simulink model "EngPrt_PrtLimMech"  (R2018a)
settings: configuration reference "cs_ert" (kept outside this file)
model workspace (MAT data in the model file):
  EngPrt_PrtLimMech_DT = 10
values from neighbouring files (symbols this model uses):
  EngPrt_facTrqLimCor_MAP = 1.0 1.0 1.0 1.0 1.0 1.0 1.0 1.0 1.0 1.0 1.0 1.0 1.0 1.0 1.0 1.0 1.0 1.0 1.0 1.0 1.0 1.0 1.0 1.0 1.0 1.0 1.0 1.0 1.0 1.0 1.0 1.0 1.0 1.0 1.0 1.0 1.0 1.0 1.0 1.0 1.0 1.0 1.0 1.0 1.0 1.0 1.0 1.0 1.0 1.0 1.0 1.0 1.0 1.0 1.0 1.0 1.0 1.0 1.0 1.0 1.0 1.0 1.0 1.0 1.0 1.0 1.0 1.0 1.0 1.0 1.0 1.0 1.0 1.0 1.0 1.0 1.0 1.0 1.0 1.0 1.0 1.0 1.0 1.0 1.0 1.0 1.0 1.0 1.0 1.0 1.0 1.0 1.0 1.0 1.0 1.0 1.0 1.0 1.0 1.0    [EngPrt_PrtLimMech.sldd]
  EngPrt_facTrqLimCor_MAPX : value not decoded    [EngPrt_PrtLimMech.sldd]
  EngPrt_facTrqLimCor_MAPY : value not decoded    [EngPrt_PrtLimMech.sldd]
  EngPrt_qLim_CUR : value not decoded    [EngPrt_PrtLimMech.sldd]
  EngPrt_qLim_CURX = 100.0 345.83333333333337 591.66666666666674 837.5 1083.3333333333335 1329.1666666666667 1575.0 1820.8333333333333 2066.666666666667 2312.5 2558.3333333333335 2804.1666666666665 3050.0 3295.8333333333335 3541.6666666666665 3787.5 4033.3333333333335 4279.166666666667 4525.0 4770.833333333333 5016.666666666667 5262.5 5508.333333333333 5754.166666666667 6000.0    [EngPrt_PrtLimMech.sldd]
  EngPrt_RmpLimNErrNeg_C = 10.0    [EngPrt_PrtLimMech.sldd]
  EngPrt_RmpLimNErrPos_C = 10.0    [EngPrt_PrtLimMech.sldd]
  EngPrt_swtLimCorType_C = 0    [EngPrt_PrtLimMech.sldd]
  EngPrt_swtTrq_C = 0.0    [EngPrt_PrtLimMech.sldd]
  EngPrt_trqLim_CUR : value not decoded    [EngPrt_PrtLimMech.sldd]
  EngPrt_trqLim_CURX : value not decoded    [EngPrt_PrtLimMech.sldd]
  EngPrt_trqLimAPSCor_MAP = 0.0 0.0 0.0 0.0 0.0 0.0 0.0 0.0 0.0 0.0 0.0 0.0 0.0 0.0 0.0 0.0 0.0 0.0 0.0 0.0 0.0 0.0 0.0 0.0 0.0 0.0 0.0 0.0 0.0 0.0 0.0 0.0 0.0 0.0 0.0 0.0 0.0 0.0 0.0 0.0 0.0 0.0 0.0 0.0 0.0 0.0 0.0 0.0 0.0 0.0 0.0 0.0 0.0 0.0 0.0 0.0 0.0 0.0 0.0 0.0 0.0 0.0 0.0 0.0 0.0 0.0 0.0 0.0 0.0 0.0 0.0 0.0 0.0 0.0 0.0 0.0 0.0 0.0 0.0 0.0 0.0 0.0 0.0 0.0 0.0 0.0 0.0 0.0 0.0 0.0 0.0 0.0 0.0 0.0 0.0 0.0 0.0 0.0 0.0 0.0    [EngPrt_PrtLimMech.sldd]
  EngPrt_trqLimAPSCor_MAPX : value not decoded    [EngPrt_PrtLimMech.sldd]
  EngPrt_trqLimAPSCor_MAPY : value not decoded    [EngPrt_PrtLimMech.sldd]
  EngPrt_trqLimEngTempCor_MAP = 0.0 0.0 0.0 0.0 0.0 0.0 0.0 0.0 0.0 0.0 0.0 0.0 0.0 0.0 0.0 0.0 0.0 0.0 0.0 0.0 0.0 0.0 0.0 0.0 0.0 0.0 0.0 0.0 0.0 0.0 0.0 0.0 0.0 0.0 0.0 0.0 0.0 0.0 0.0 0.0 0.0 0.0 0.0 0.0 0.0 0.0 0.0 0.0 0.0 0.0 0.0 0.0 0.0 0.0 0.0 0.0 0.0 0.0 0.0 0.0 0.0 0.0 0.0 0.0 0.0 0.0 0.0 0.0 0.0 0.0 0.0 0.0 0.0 0.0 0.0 0.0 0.0 0.0 0.0 0.0 0.0 0.0 0.0 0.0 0.0 0.0 0.0 0.0 0.0 0.0 0.0 0.0 0.0 0.0 0.0 0.0 0.0 0.0 0.0 0.0    [EngPrt_PrtLimMech.sldd]
  EngPrt_trqLimEngTempCor_MAPX : value not decoded    [EngPrt_PrtLimMech.sldd]
  EngPrt_trqLimEngTempCor_MAPY : value not decoded    [EngPrt_PrtLimMech.sldd]
  EngPrt_trqNLim_CUR : value not decoded    [EngPrt_PrtLimMech.sldd]
  EngPrt_trqNLim_CURX : value not decoded    [EngPrt_PrtLimMech.sldd]
  EngPrt_trqNLimSpr_CUR : value not decoded    [EngPrt_PrtLimMech.sldd]
  EngPrt_trqNLimSpr_CURX : value not decoded    [EngPrt_PrtLimMech.sldd]
undefined symbols (not defined in the file or in its folder): Switch
libraries: sllib x1
settings Model: DataDictionary=EngPrt_PrtLimMech.sldd  Creator=zhoutinglin  LastModifiedBy=zhoutinglin

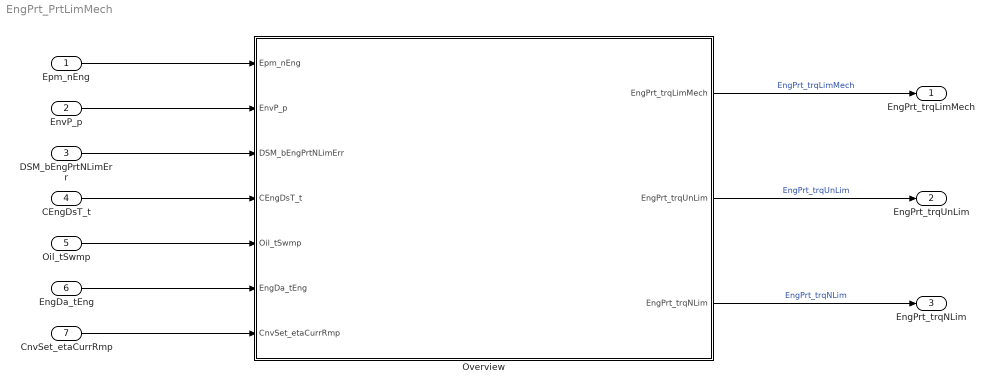
== system EngPrt_PrtLimMech ==
  Epm_nEng : Inport  Description=Engine speed  OutMin=0  OutMax=6000  OutDataTypeStr=ERPM  Unit=rpm  PortDimensions=[1 1]
  EnvP_p : Inport  Description=Barometric pressure  Port=2  OutMin=0  OutMax=300  OutDataTypeStr=Press_kpa  Unit=kPa  PortDimensions=[1 1]
  DSM_bEngPrtNLimErr : Inport  Description=Activation of additional engine speed limitation  Port=3  OutMin=0  OutMax=1  OutDataTypeStr=boolean  PortDimensions=[1 1]
  CEngDsT_t : Inport  Description=engine coolant temperature after filter  Port=4  OutMin=-200  OutMax=200  OutDataTypeStr=Temp_C  Unit=deg  PortDimensions=[1 1]
  Oil_tSwmp : Inport  Description=Oil temperature in oil sump  Port=5  OutMin=-50  OutMax=200  OutDataTypeStr=Temp_C  Unit=deg  PortDimensions=[1 1]
  EngDa_tEng : Inport  Description=Engine temperature  Port=6  OutMin=-1000  OutMax=1000  OutDataTypeStr=Temp_C  Unit=deg  PortDimensions=[1 1]
  CnvSet_etaCurrRmp : Inport  Description=Conversion efficiency corresponding to CnvSet_qSet  Port=7  OutMin=0  OutMax=100  OutDataTypeStr=Effcy  Unit=Nm/(mg/hub)  PortDimensions=[1 1]
  Overview : Subsystem
  EngPrt_trqLimMech : Outport
  EngPrt_trqUnLim : Outport  Port=2
  EngPrt_trqNLim : Outport  Port=3
  wires:
  Epm_nEng/1 -> Overview/1(Epm_nEng)
  EnvP_p/1 -> Overview/2(EnvP_p)
  DSM_bEngPrtNLimErr/1 -> Overview/3(DSM_bEngPrtNLimErr)
  CEngDsT_t/1 -> Overview/4(CEngDsT_t)
  Oil_tSwmp/1 -> Overview/5(Oil_tSwmp)
  EngDa_tEng/1 -> Overview/6(EngDa_tEng)
  CnvSet_etaCurrRmp/1 -> Overview/7(CnvSet_etaCurrRmp)
  Overview/1(EngPrt_trqLimMech) -> EngPrt_trqLimMech/1  "EngPrt_trqLimMech"
  Overview/2(EngPrt_trqUnLim) -> EngPrt_trqUnLim/1  "EngPrt_trqUnLim"
  Overview/3(EngPrt_trqNLim) -> EngPrt_trqNLim/1  "EngPrt_trqNLim"

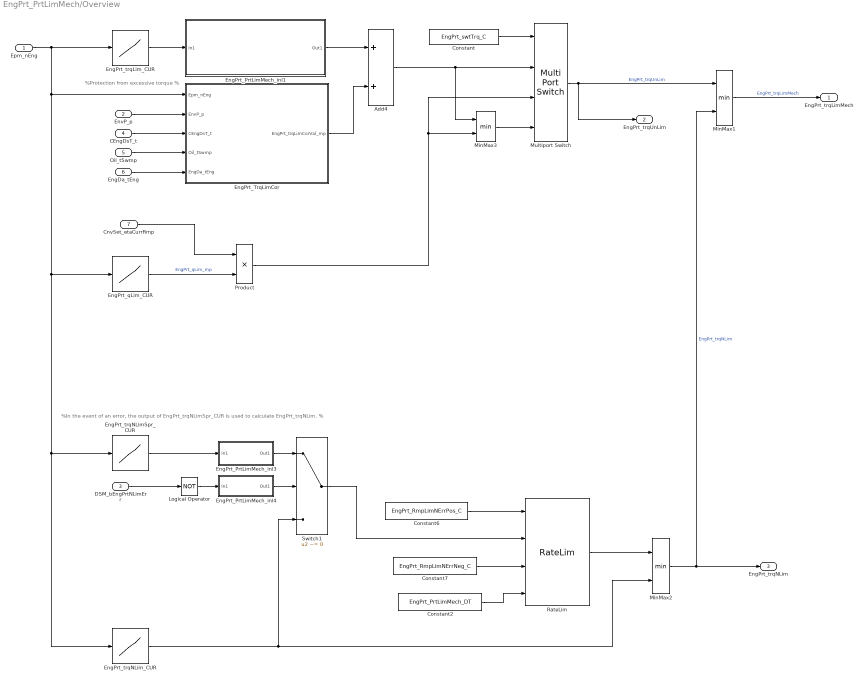
== system EngPrt_PrtLimMech/Overview ==
  note: %Protection from excessive torque %
  note: %In the event of an error, the output of EngPrt_trqNLimSpr_CUR is used to calculate EngPrt_trqNLim. %
  Epm_nEng : Inport  Tag=rpm
  EnvP_p : Inport  Tag=kPa  Port=2
  DSM_bEngPrtNLimErr : Inport  Port=3
  CEngDsT_t : Inport  Tag=deg  Port=4
  Oil_tSwmp : Inport  Tag=deg  Port=5
  EngDa_tEng : Inport  Tag=deg  Port=6
  CnvSet_etaCurrRmp : Inport  Tag=Nm/(mg/hub)  Port=7
  Add4 : Sum  InputSameDT=on
  Constant : Constant  Value=EngPrt_swtTrq_C
  Constant2 : Constant  Value=EngPrt_PrtLimMech_DT  OutDataTypeStr=Inherit: Inherit via back propagation
  Constant6 : Constant  Value=EngPrt_RmpLimNErrPos_C
  Constant7 : Constant  Value=EngPrt_RmpLimNErrNeg_C
  EngPrt_PrtLimMech_inl1 : Subsystem
  EngPrt_PrtLimMech_inl3 : Subsystem
  EngPrt_PrtLimMech_inl4 : Subsystem
  EngPrt_TrqLimCor : Subsystem
  EngPrt_qLim_CUR : Lookup_n-D  NumberOfTableDimensions=1  BreakpointsForDimension1=EngPrt_qLim_CURX  BreakpointsForDimension2=[1:3]  IndexSearchMethod=Linear search  Table=EngPrt_qLim_CUR  ExtrapMethod=Clip  InternalRulePriority=Speed  OutDataTypeStr=Inherit: Inherit via back propagation  RndMeth=Simplest  SaturateOnIntegerOverflow=on
  EngPrt_trqLim_CUR : Lookup_n-D  NumberOfTableDimensions=1  BreakpointsForDimension1=EngPrt_trqLim_CURX  BreakpointsForDimension2=[1:3]  IndexSearchMethod=Linear search  Table=EngPrt_trqLim_CUR  ExtrapMethod=Clip  InternalRulePriority=Speed  OutDataTypeStr=Inherit: Inherit via back propagation  RndMeth=Simplest  SaturateOnIntegerOverflow=on
  EngPrt_trqNLimSpr_CUR : Lookup_n-D  NumberOfTableDimensions=1  BreakpointsForDimension1=EngPrt_trqNLimSpr_CURX  BreakpointsForDimension2=[1:3]  IndexSearchMethod=Linear search  Table=EngPrt_trqNLimSpr_CUR  ExtrapMethod=Clip  InternalRulePriority=Speed  OutDataTypeStr=Inherit: Inherit via back propagation  RndMeth=Simplest  SaturateOnIntegerOverflow=on
  EngPrt_trqNLim_CUR : Lookup_n-D  NumberOfTableDimensions=1  BreakpointsForDimension1=EngPrt_trqNLim_CURX  BreakpointsForDimension2=[1:3]  IndexSearchMethod=Linear search  Table=EngPrt_trqNLim_CUR  ExtrapMethod=Clip  InternalRulePriority=Speed  OutDataTypeStr=Inherit: Inherit via back propagation  RndMeth=Simplest  SaturateOnIntegerOverflow=on
  Logical Operator : Logic  Operator=NOT  AllPortsSameDT=off  OutDataTypeStr=boolean
  MinMax1 : MinMax  Inputs=2  InputSameDT=on
  MinMax2 : MinMax  Inputs=2  InputSameDT=on
  MinMax3 : MinMax  Inputs=2  InputSameDT=on
  Multiport Switch : MultiPortSwitch  DataPortOrder=Zero-based contiguous  zeroidx=on  OutDataTypeStr=Inherit: Inherit via back propagation  InputSameDT=on
  Product : Product  OutDataTypeStr=Inherit: Inherit via back propagation  SaturateOnIntegerOverflow=on
  RateLim : sllib/RateLim
      settings: SourceProductName=sllib
  Switch1 : Switch  Criteria=u2 ~= 0  InputSameDT=on
  EngPrt_trqLimMech : Outport  Tag=Nm
  EngPrt_trqUnLim : Outport  Tag=Nm  Port=2
  EngPrt_trqNLim : Outport  Tag=Nm  Port=3
  wires:
  Add4/1 -> Multiport Switch/2, MinMax3/1
  Multiport Switch/1 -> EngPrt_trqUnLim/1, MinMax1/1  "EngPrt_trqUnLim"
  EngPrt_trqNLim_CUR/1 -> MinMax2/2, Switch1/3
  CnvSet_etaCurrRmp/1 -> Product/1
  EngPrt_qLim_CUR/1 -> Product/2  "EngPrt_qLim_mp"
  Product/1 -> Multiport Switch/3, MinMax3/2
  MinMax2/1 -> MinMax1/2, EngPrt_trqNLim/1  "EngPrt_trqNLim"
  RateLim/1 -> MinMax2/1
  Constant2/1 -> RateLim/4
  Constant/1 -> Multiport Switch/1
  EngPrt_PrtLimMech_inl4/1(Out1) -> Switch1/2
  MinMax3/1 -> Multiport Switch/4
  Oil_tSwmp/1 -> EngPrt_TrqLimCor/4(Oil_tSwmp)
  EngPrt_PrtLimMech_inl1/1(Out1) -> Add4/1
  MinMax1/1 -> EngPrt_trqLimMech/1  "EngPrt_trqLimMech"
  EngPrt_trqNLimSpr_CUR/1 -> EngPrt_PrtLimMech_inl3/1(In1)
  DSM_bEngPrtNLimErr/1 -> Logical Operator/1
  Switch1/1 -> RateLim/2
  EngPrt_PrtLimMech_inl3/1(Out1) -> Switch1/1
  Constant7/1 -> RateLim/3
  Constant6/1 -> RateLim/1
  EngDa_tEng/1 -> EngPrt_TrqLimCor/5(EngDa_tEng)
  EngPrt_TrqLimCor/1(EngPrt_trqLimCorVal_mp) -> Add4/2
  EnvP_p/1 -> EngPrt_TrqLimCor/2(EnvP_p)
  CEngDsT_t/1 -> EngPrt_TrqLimCor/3(CEngDsT_t)
  Logical Operator/1 -> EngPrt_PrtLimMech_inl4/1(In1)
  EngPrt_trqLim_CUR/1 -> EngPrt_PrtLimMech_inl1/1(In1)
  Epm_nEng/1 -> EngPrt_qLim_CUR/1, EngPrt_trqNLim_CUR/1, EngPrt_trqNLimSpr_CUR/1, EngPrt_TrqLimCor/1(Epm_nEng), EngPrt_trqLim_CUR/1

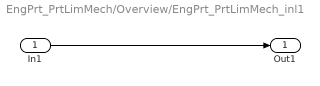
== system EngPrt_PrtLimMech/Overview/EngPrt_PrtLimMech_inl1 ==
  In1 : Inport
  Out1 : Outport
  wires:
  In1/1 -> Out1/1

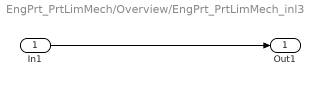
== system EngPrt_PrtLimMech/Overview/EngPrt_PrtLimMech_inl3 ==
  In1 : Inport
  Out1 : Outport
  wires:
  In1/1 -> Out1/1

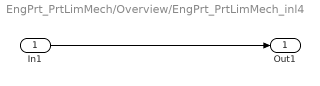
== system EngPrt_PrtLimMech/Overview/EngPrt_PrtLimMech_inl4 ==
  In1 : Inport
  Out1 : Outport
  wires:
  In1/1 -> Out1/1

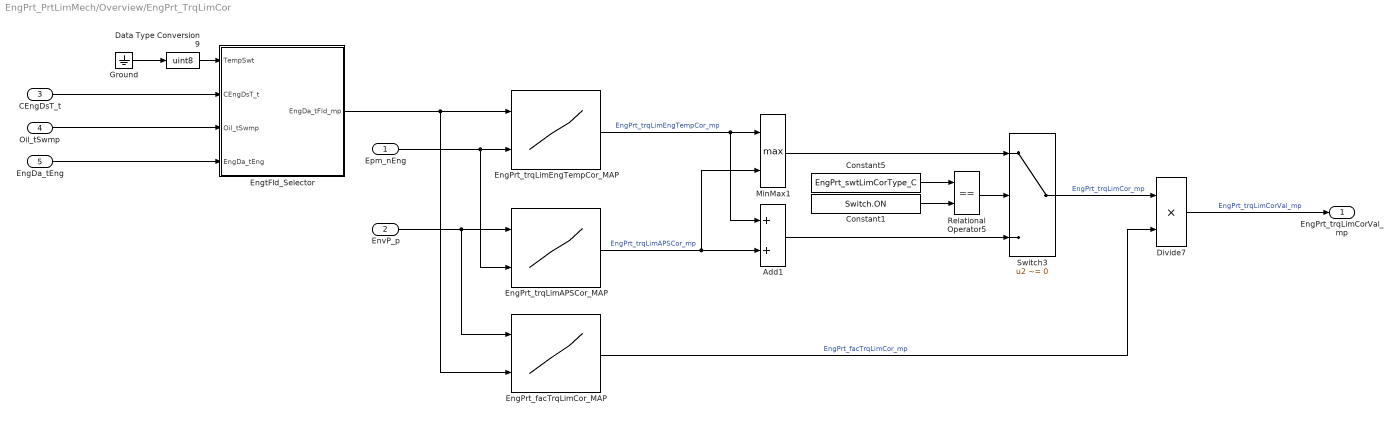
== system EngPrt_PrtLimMech/Overview/EngPrt_TrqLimCor ==
  Epm_nEng : Inport
  EnvP_p : Inport  Port=2
  CEngDsT_t : Inport  Tag=deg  Port=3
  Oil_tSwmp : Inport  Tag=deg  Port=4
  EngDa_tEng : Inport  Tag=deg  Port=5
  Add1 : Sum  InputSameDT=on
  Constant1 : Constant  Value=Switch.ON  OutDataTypeStr=Inherit: Inherit via back propagation
  Constant5 : Constant  Value=EngPrt_swtLimCorType_C
  Data Type Conversion9 : DataTypeConversion  OutDataTypeStr=uint8
  Divide7 : Product  Inputs=**  OutDataTypeStr=Inherit: Inherit via back propagation
  EngPrt_facTrqLimCor_MAP : Lookup_n-D  DialogController=Simulink.DDGSource  BreakpointsForDimension1=EngPrt_facTrqLimCor_MAPY  BreakpointsForDimension2=EngPrt_facTrqLimCor_MAPX  BreakpointsForDimension1DataTypeStr=Inherit: Inherit from 'Breakpoint data'  BreakpointsForDimension2DataTypeStr=Inherit: Inherit from 'Breakpoint data'  BeginIndexSearchUsingPreviousIndexResult=on  Table=EngPrt_facTrqLimCor_MAP  TableDataTypeStr=Inherit: Inherit from 'Table data'  ExtrapMethod=Clip  UseLastTableValue=on  InternalRulePriority=Speed  OutDataTypeStr=Inherit: Inherit from 'Table data'  SaturateOnIntegerOverflow=on
  EngPrt_trqLimAPSCor_MAP : Lookup_n-D  DialogController=Simulink.DDGSource  BreakpointsForDimension1=EngPrt_trqLimAPSCor_MAPY  BreakpointsForDimension2=EngPrt_trqLimAPSCor_MAPX  IndexSearchMethod=Linear search  BeginIndexSearchUsingPreviousIndexResult=on  Table=EngPrt_trqLimAPSCor_MAP  ExtrapMethod=Clip  UseLastTableValue=on  InternalRulePriority=Speed  OutDataTypeStr=Inherit: Inherit via back propagation  SaturateOnIntegerOverflow=on
  EngPrt_trqLimEngTempCor_MAP : Lookup_n-D  DialogController=Simulink.DDGSource  BreakpointsForDimension1=EngPrt_trqLimEngTempCor_MAPY  BreakpointsForDimension2=EngPrt_trqLimEngTempCor_MAPX  IndexSearchMethod=Linear search  BeginIndexSearchUsingPreviousIndexResult=on  Table=EngPrt_trqLimEngTempCor_MAP  ExtrapMethod=Clip  UseLastTableValue=on  InternalRulePriority=Speed  OutDataTypeStr=Inherit: Inherit via back propagation  SaturateOnIntegerOverflow=on
  EngtFld_Selector : Subsystem
  Ground : Ground
  MinMax1 : MinMax  Function=max  Inputs=2  InputSameDT=on
  Relational Operator5 : RelationalOperator  Operator===  OutDataTypeStr=boolean  RndMeth=Simplest  InputSameDT=on
  Switch3 : Switch  Criteria=u2 ~= 0  InputSameDT=on
  EngPrt_trqLimCorVal_mp : Outport
  wires:
  Constant1/1 -> Relational Operator5/2
  Relational Operator5/1 -> Switch3/2
  Epm_nEng/1 -> EngPrt_trqLimAPSCor_MAP/2, EngPrt_trqLimEngTempCor_MAP/2
  EngtFld_Selector/1(EngDa_tFld_mp) -> EngPrt_facTrqLimCor_MAP/2, EngPrt_trqLimEngTempCor_MAP/1
  EnvP_p/1 -> EngPrt_facTrqLimCor_MAP/1, EngPrt_trqLimAPSCor_MAP/1
  EngPrt_facTrqLimCor_MAP/1 -> Divide7/2  "EngPrt_facTrqLimCor_mp"
  EngPrt_trqLimAPSCor_MAP/1 -> MinMax1/2, Add1/2  "EngPrt_trqLimAPSCor_mp"
  EngPrt_trqLimEngTempCor_MAP/1 -> Add1/1, MinMax1/1  "EngPrt_trqLimEngTempCor_mp"
  Add1/1 -> Switch3/3
  MinMax1/1 -> Switch3/1
  Constant5/1 -> Relational Operator5/1
  Divide7/1 -> EngPrt_trqLimCorVal_mp/1  "EngPrt_trqLimCorVal_mp"
  Switch3/1 -> Divide7/1  "EngPrt_trqLimCor_mp"
  Ground/1 -> Data Type Conversion9/1
  Data Type Conversion9/1 -> EngtFld_Selector/1(TempSwt)
  CEngDsT_t/1 -> EngtFld_Selector/2(CEngDsT_t)
  Oil_tSwmp/1 -> EngtFld_Selector/3(Oil_tSwmp)
  EngDa_tEng/1 -> EngtFld_Selector/4(EngDa_tEng)

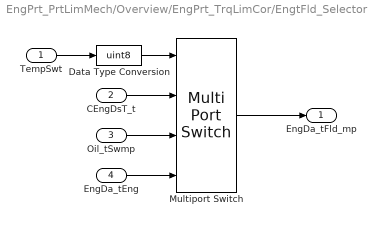
== system EngPrt_PrtLimMech/Overview/EngPrt_TrqLimCor/EngtFld_Selector ==
  TempSwt : Inport
  CEngDsT_t : Inport  Tag=deg  Port=2
  Oil_tSwmp : Inport  Tag=deg  Port=3
  EngDa_tEng : Inport  Tag=deg  Port=4
  Data Type Conversion : DataTypeConversion  OutDataTypeStr=uint8
  Multiport Switch : MultiPortSwitch  DataPortOrder=Zero-based contiguous  zeroidx=on
  EngDa_tFld_mp : Outport  Tag=deg
  wires:
  CEngDsT_t/1 -> Multiport Switch/2
  Multiport Switch/1 -> EngDa_tFld_mp/1
  EngDa_tEng/1 -> Multiport Switch/4
  Oil_tSwmp/1 -> Multiport Switch/3
  Data Type Conversion/1 -> Multiport Switch/1
  TempSwt/1 -> Data Type Conversion/1
